simulink model "part3_LQR2_sim"  (R2017a)
settings: Solver=VariableStepAuto  StartTime=0.0  StopTime=simTime  RelTol=1e-3
values from neighbouring files (symbols this model uses):
  A = [0 0 0 0 0 0 40.7055790872 38.6368253303 1 0 -13.2363115295 -4.71950452077 ... (16 elements, 4x4)]    [model.mat]    (also in part1_lin_model.m = [)
  B = [0 0 23.29957643 8.30763585823]    [model.mat]    (also in part1_lin_model.m = [)
  C = [1  0  0  0; 0  1  0  0]    [model.mat]    (also in part1_lin_model.m = eye(2,4))
  D = [0 0]    [model.mat]    (also in part1_lin_model.m = zeros(2,1))
  Omgc = fc*(2*pi)    (= 50.2654824574)    [part3_designController.m]    (also in part4.m = 12.5663706144)
  theta_d = 1    [part2_designController.m]    (also in part3_designController.m = -0.785398163397; part4.m)
  Ts = 1/200    (= 0.005)    [part2_designController.m]    (also in part3_designController.m; part4.m)
  x0 = [0;0;0;0]    [part2_designController.m]    (also in part3_designController.m; part4.m)
undefined symbols (not defined in the file or in its folder): K
settings Model: Creator=zilleplus  LastModifiedBy=zilleplus

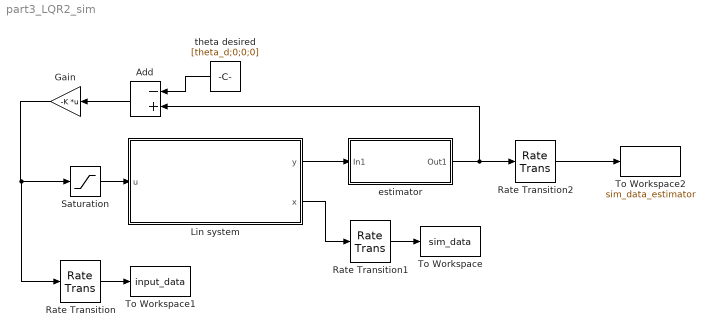
== system part3_LQR2_sim ==
  Add : Sum  Inputs=-+
  Gain : Gain  Gain=-K  Multiplication=Matrix(K*u) (u vector)
  Lin system : Subsystem
  Rate Transition : RateTransition
  Rate Transition1 : RateTransition  OutPortSampleTime=Ts
  Rate Transition2 : RateTransition  OutPortSampleTime=Ts
  Saturation : Saturate  UpperLimit=5  LowerLimit=-5
  To Workspace : ToWorkspace  VariableName=sim_data  SaveFormat=Timeseries  SampleTime=-1
  To Workspace1 : ToWorkspace  VariableName=input_data  SaveFormat=Timeseries  SampleTime=Ts
  To Workspace2 : ToWorkspace  VariableName=sim_data_estimator  SaveFormat=Timeseries  SampleTime=Ts
  estimator : Subsystem
  theta desired : Constant  Value=[theta_d;0;0;0]
  wires:
  Gain/1 -> Rate Transition/1, Saturation/1
  Lin system/2(x) -> Rate Transition1/1
  Add/1 -> Gain/1
  Saturation/1 -> Lin system/1(u)
  theta desired/1 -> Add/1
  Rate Transition/1 -> To Workspace1/1
  Rate Transition1/1 -> To Workspace/1
  Lin system/1(y) -> estimator/1(In1)
  estimator/1(Out1) -> Rate Transition2/1, Add/2
  Rate Transition2/1 -> To Workspace2/1

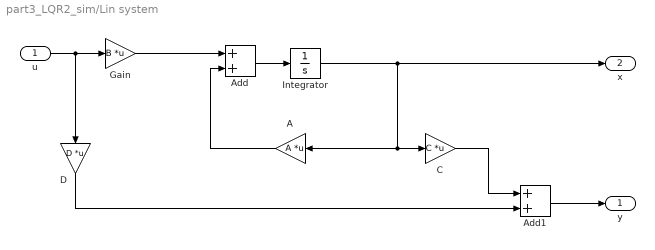
== system part3_LQR2_sim/Lin system ==
  u : Inport
  A : Gain  Gain=A  Multiplication=Matrix(K*u) (u vector)
  Add : Sum
  Add1 : Sum
  C : Gain  Gain=C  Multiplication=Matrix(K*u) (u vector)
  D : Gain  Gain=D  Multiplication=Matrix(K*u) (u vector)
  Gain : Gain  Gain=B  Multiplication=Matrix(K*u) (u vector)
  Integrator : Integrator  InitialCondition=x0
  y : Outport
  x : Outport  Port=2
  wires:
  u/1 -> D/1, Gain/1
  Integrator/1 -> x/1, A/1, C/1
  A/1 -> Add/2
  Gain/1 -> Add/1
  C/1 -> Add1/1
  Add1/1 -> y/1
  D/1 -> Add1/2
  Add/1 -> Integrator/1

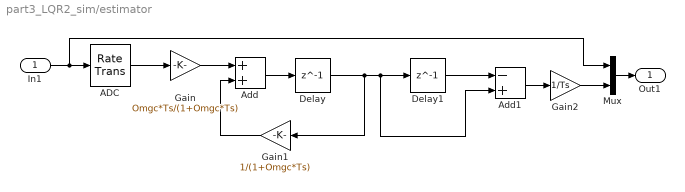
== system part3_LQR2_sim/estimator ==
  In1 : Inport
  "ADC " : RateTransition  OutPortSampleTime=Ts
  Add : Sum
  Add1 : Sum  Inputs=-+
  Delay : Delay  DelayLength=1  InitialCondition=0
  Delay1 : Delay  DelayLength=1  InitialCondition=0
  Gain : Gain  Gain=Omgc*Ts/(1+Omgc*Ts)
  Gain1 : Gain  Gain=1/(1+Omgc*Ts)
  Gain2 : Gain  Gain=1/Ts
  Mux : Mux  Inputs=2
  Out1 : Outport
  wires:
  In1/1 -> Mux/1, "ADC "/1
  "ADC "/1 -> Gain/1
  Delay/1 -> Add1/2, Delay1/1, Gain1/1
  Gain/1 -> Add/1
  Add/1 -> Delay/1
  Gain1/1 -> Add/2
  Delay1/1 -> Add1/1
  Mux/1 -> Out1/1
  Add1/1 -> Gain2/1
  Gain2/1 -> Mux/2
